simulink model "animation"  (R2020a)
settings: Solver=ode8  StartTime=0.0  StopTime=3600  FixedStep=1  RelTol=1e-3
libraries: vrlib x7, sharedtransform x3, simulink x1
settings Model: Creator=bbingham  LastModifiedBy=bbingham
settings DataIOCC: SaveOutput=off  SignalLogging=off  DSMLogging=off  SaveTime=off  ReturnWorkspaceOutputs=off
settings DebuggingCC: ArithmeticOperatorsInVariantConditions=warning
settings SFSimCC: SimUseLocalCustomCode=off  CustomCodeUndefinedFunction=UseInterfaceOnly
settings RTWCC: RTWUseLocalCustomCode=off
settings CodeAppCC: StateflowObjectComments=on

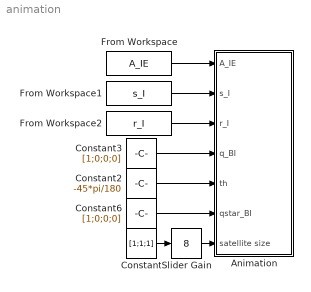
== system animation ==
  Animation : Subsystem
  Constant : Constant  Value=[1;1;1]
  Constant2 : Constant  Value=-45*pi/180
  Constant3 : Constant  Value=[1;0;0;0]
  Constant6 : Constant  Value=[1;0;0;0]
  From Workspace : FromWorkspace  VariableName=A_IE
  From Workspace1 : FromWorkspace  VariableName=s_I
  From Workspace2 : FromWorkspace  VariableName=r_I
  Slider Gain : simulink/Math Operations/Slider Gain  gain=8  low=1  high=50
  wires:
  Constant2/1 -> Animation/5(th)
  Constant/1 -> Slider Gain/1
  Slider Gain/1 -> Animation/7(satellite size)
  Constant6/1 -> Animation/6(qstar_BI)
  Constant3/1 -> Animation/4(q_BI)
  From Workspace/1 -> Animation/1(A_IE)
  From Workspace1/1 -> Animation/2(s_I)
  From Workspace2/1 -> Animation/3(r_I)

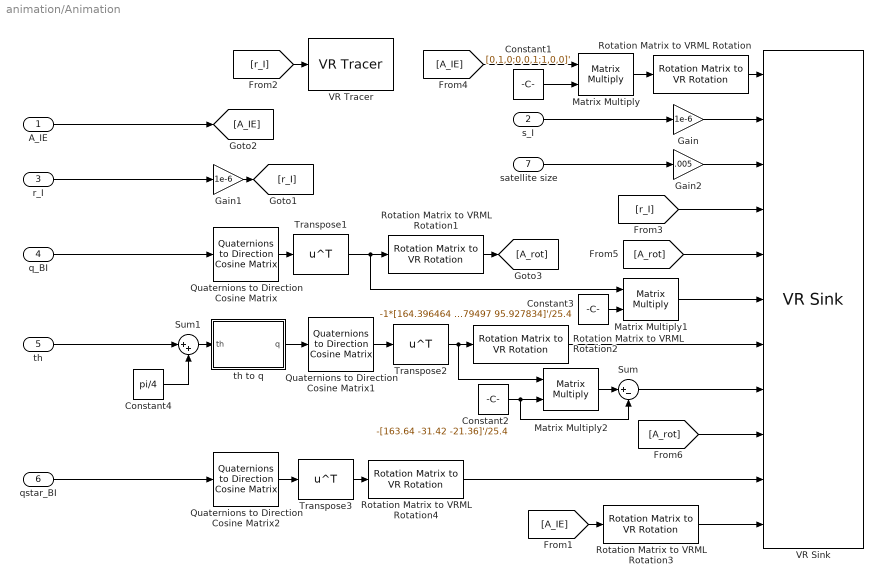
== system animation/Animation ==
  A_IE : Inport
  s_I : Inport  Port=2
  r_I : Inport  Port=3
  q_BI : Inport  Port=4
  th : Inport  Port=5
  qstar_BI : Inport  Port=6
  satellite size : Inport  Port=7
  Constant1 : Constant  Value=[0,1,0;0,0,1;1,0,0]'
  Constant2 : Constant  Value=-[163.64 -31.42 -21.36]'/25.4
  Constant3 : Constant  Value=-1*[164.396464 -81.879497 95.927834]'/25.4
  Constant4 : Constant  Value=pi/4
  Gain : Gain  Gain=1e-6
  Gain1 : Gain  Gain=1e-6
  Gain2 : Gain  Gain=.005
  Matrix Multiply : Product  Multiplication=Matrix(*)
  Matrix Multiply1 : Product  Multiplication=Matrix(*)
  Matrix Multiply2 : Product  Multiplication=Matrix(*)
  Quaternions to Direction Cosine Matrix : sharedtransform/Quaternions to  Direction Cosine Matrix  aMode=aMode
      settings: SourceProductBaseCode=AE,PW,MT,VE,VP
  Quaternions to Direction Cosine Matrix1 : sharedtransform/Quaternions to  Direction Cosine Matrix  aMode=aMode
      settings: SourceProductBaseCode=AE,PW,MT,VE,VP
  Quaternions to Direction Cosine Matrix2 : sharedtransform/Quaternions to  Direction Cosine Matrix  aMode=aMode
      settings: SourceProductBaseCode=AE,PW,MT,VE,VP
  Rotation Matrix to VRML Rotation{,1..4} (5 alike) : vrlib/Utilities/Rotation Matrix to VR Rotation  maxzero=1e-12
      settings: SourceProductBaseCode=SL
  Sum : Sum  Inputs=|+-
  Sum1 : Sum  Inputs=|++
  Transpose1 : Math  Operator=transpose  SignedPower=on  SaturateOnIntegerOverflow=on
  Transpose2 : Math  Operator=transpose  SignedPower=on  SaturateOnIntegerOverflow=on
  Transpose3 : Math  Operator=transpose  SignedPower=on  SaturateOnIntegerOverflow=on
  VR Sink : vrlib/VR Sink  InstantiateOnLoad=on  SampleTime=2  ViewEnable=on  RemoteChange=off  RemoteView=off  FieldsWritten=Earth.rotation.4.1.1.double#Sun.translation.3.1.1.double#Satellite.scale.3.1.1.double#Satellite.translation.3.1.1.double#Chassis.rotation.4.1.1.double#Chassis.translation.3.1.1.double#Panel.rotation.4.1.1.double#Panel.translation.3.1.1.double#Body_Axes.rotation.4.1.1.double#Target_Axes.rotation.4.1.1.double#ECEF_Axes.rotation.4.1.1.double  WorldFileName=earth.wrl  WorldDescription=Orbital Animation  AutoView=on  VideoDimensions=[]  AllowVariableSize=off
  VR Tracer : vrlib/VR Tracer  VrmlFile=earth.wrl  MarkerName=None  UseLines=on  UseTriads=off  MarkerScale=[1 1 1]  MarkerColorSelection=Selected from color list  MarkerColor=magenta  rgbval=[1 0 0]  Ts=-1  ForceViewerOpen=off  ConnectPlane=off  PlaneCoeff=[0 1 0 0]  ConnectPoint=None  PointCoord=[0 0 0]
      settings: SourceProductBaseCode=SL
  th to q : MATLAB Function  TreatAsAtomicUnit=on
  wires:
  Constant1/1 -> Matrix Multiply/2
  Quaternions to Direction Cosine Matrix/1 -> Transpose1/1
  Transpose1/1 -> Matrix Multiply1/1, Rotation Matrix to VRML Rotation1/1
  Constant3/1 -> Matrix Multiply1/2
  th to q/1(q) -> Quaternions to Direction Cosine Matrix1/1
  Quaternions to Direction Cosine Matrix1/1 -> Transpose2/1
  Transpose2/1 -> Rotation Matrix to VRML Rotation2/1, Matrix Multiply2/1
  Constant2/1 -> Matrix Multiply2/2, Sum/2
  Matrix Multiply2/1 -> Sum/1
  Quaternions to Direction Cosine Matrix2/1 -> Transpose3/1
  Transpose3/1 -> Rotation Matrix to VRML Rotation4/1
  [A_IE] -> Rotation Matrix to VRML Rotation3/1
  Gain1/1 -> [r_I]
  Rotation Matrix to VRML Rotation1/1 -> [A_rot]
  Sum1/1 -> th to q/1(th)
  Constant4/1 -> Sum1/2
  Rotation Matrix to VRML Rotation/1 -> VR Sink/1
  Gain/1 -> VR Sink/2
  Gain2/1 -> VR Sink/3
  [r_I] -> VR Sink/4
  [A_rot] -> VR Sink/5
  Matrix Multiply1/1 -> VR Sink/6
  Rotation Matrix to VRML Rotation2/1 -> VR Sink/7
  Sum/1 -> VR Sink/8
  [A_rot] -> VR Sink/9
  Rotation Matrix to VRML Rotation4/1 -> VR Sink/10
  Rotation Matrix to VRML Rotation3/1 -> VR Sink/11
  [r_I] -> VR Tracer/1
  A_IE/1 -> [A_IE]
  r_I/1 -> Gain1/1
  q_BI/1 -> Quaternions to Direction Cosine Matrix/1
  th/1 -> Sum1/1
  qstar_BI/1 -> Quaternions to Direction Cosine Matrix2/1
  s_I/1 -> Gain/1
  satellite size/1 -> Gain2/1
  [A_IE] -> Matrix Multiply/1
  Matrix Multiply/1 -> Rotation Matrix to VRML Rotation/1

== matlab function animation/Animation/th to q ==
  data: th input; q output
function q = fcn(th)
%#codegen

q = [cos(th/2);sin(th/2);0;0];
